simulink model "Crane_LQR_realSetup2016_obnoxious"  (R2016b)
settings: Solver=VariableStepAuto  StartTime=0.0  StopTime=30  RelTol=1e-3
undefined symbols (not defined in the file): adinchannels, adinchannelsencoders, adingain, adingainencoders, adinoffs, adinoffsencoders, Ao, Bo, Co, daoutchannels, daoutgain, daoutoffs, Discrete, Do, F, h, Humusoft, MF634, RefFWD, sigbuilder_block, Time, Ts
libraries: sldrtlib x3, dspfdesign x2, ctrlSharedLib x1
settings Model: Creator=tcbooij  LastModifiedBy=tcbooij

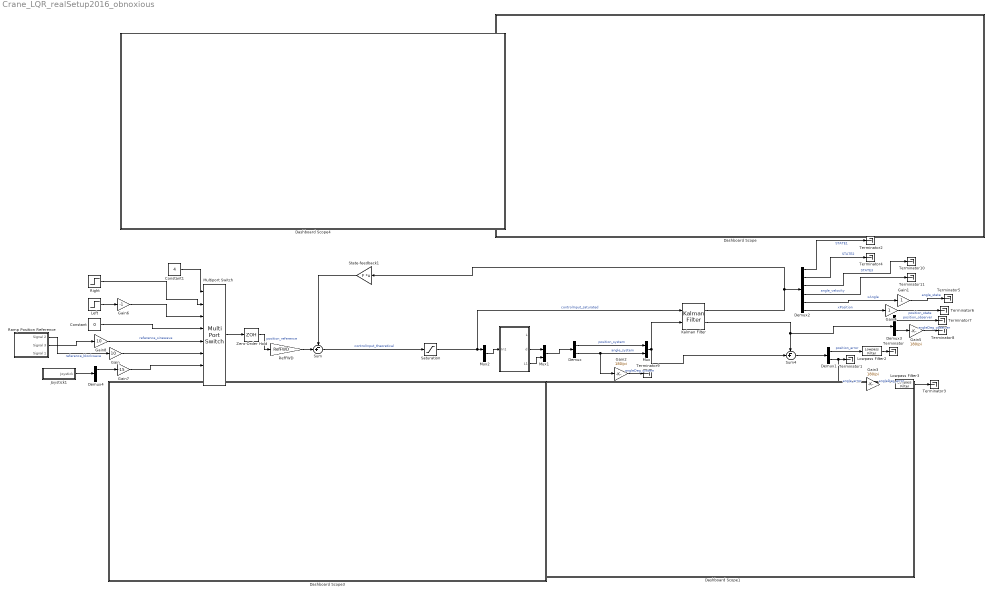
== system Crane_LQR_realSetup2016_obnoxious ==
  " " : Subsystem  LoadFcn=hwinit  InitFcn=hwinit  mask{h=h}
      mask prompts: h "Sampling period [s]"
      mask Display: disp('Crane')
  Constant : Constant  Value=0
  Constant1 : Constant  Value=4
  Dashboard Scope : Subsystem  DialogController=hmiCreateDDGDialog  IsWebBlock=on  mask(MWDashboardBlock){webBlockId=9ceaf0bf-3731-4580-b602-55a798613066, webBlockType=sdiscope, ShowInitialText=on, HMISrcModelName=Crane_LQR_realSetup2016_obnoxious}
      mask prompts: webBlockId "WebBlock Id"; webBlockType "WebBlock Type"; HMISrcModelName "Source Model"
      mask help: SimulinkHMI:dialogs:HMIScopeDialogDesc
      mask Help: helpview([docroot '/mapfiles/simulink.map'], 'hmi_scope')
      mask Display:
      | if strcmp(get_param(bdroot(gcb),'BlockDiagramType'), 'library')
      |     image([(matlabroot) '/toolbox/simulink/hmi/icons/DashboardScope.png']);
      | end
  Dashboard Scope1 : Subsystem  DialogController=hmiCreateDDGDialog  IsWebBlock=on  mask(MWDashboardBlock){webBlockId=94ce42f8-c4e1-41da-82c1-a31c02963333, webBlockType=sdiscope, ShowInitialText=on, HMISrcModelName=Crane_LQR_realSetup2016_obnoxious}
      mask prompts: webBlockId "WebBlock Id"; webBlockType "WebBlock Type"; HMISrcModelName "Source Model"
      mask help: SimulinkHMI:dialogs:HMIScopeDialogDesc
      mask Help: helpview([docroot '/mapfiles/simulink.map'], 'hmi_scope')
      mask Display:
      | if strcmp(get_param(bdroot(gcb),'BlockDiagramType'), 'library')
      |     image([(matlabroot) '/toolbox/simulink/hmi/icons/DashboardScope.png']);
      | end
  Dashboard Scope3 : Subsystem  DialogController=hmiCreateDDGDialog  IsWebBlock=on  mask(MWDashboardBlock){webBlockId=8652e169-738a-43eb-99bc-869d98056901, webBlockType=sdiscope, ShowInitialText=on, HMISrcModelName=Crane_LQR_realSetup2016_obnoxious}
      mask prompts: webBlockId "WebBlock Id"; webBlockType "WebBlock Type"; HMISrcModelName "Source Model"
      mask help: SimulinkHMI:dialogs:HMIScopeDialogDesc
      mask Help: helpview([docroot '/mapfiles/simulink.map'], 'hmi_scope')
      mask Display:
      | if strcmp(get_param(bdroot(gcb),'BlockDiagramType'), 'library')
      |     image([(matlabroot) '/toolbox/simulink/hmi/icons/DashboardScope.png']);
      | end
  Dashboard Scope4 : Subsystem  DialogController=hmiCreateDDGDialog  IsWebBlock=on  mask(MWDashboardBlock){webBlockId=041abe84-c255-4045-9a48-2957c8828250, webBlockType=sdiscope, ShowInitialText=on, HMISrcModelName=Crane_LQR_realSetup2016_obnoxious}
      mask prompts: webBlockId "WebBlock Id"; webBlockType "WebBlock Type"; HMISrcModelName "Source Model"
      mask help: SimulinkHMI:dialogs:HMIScopeDialogDesc
      mask Help: helpview([docroot '/mapfiles/simulink.map'], 'hmi_scope')
      mask Display:
      | if strcmp(get_param(bdroot(gcb),'BlockDiagramType'), 'library')
      |     image([(matlabroot) '/toolbox/simulink/hmi/icons/DashboardScope.png']);
      | end
  Demux{,1,3..4} (4 alike) : Demux  Outputs=2
  Demux2 : Demux  Outputs=6
  Gain : Gain  Gain=10
  Gain1 : Gain
  Gain2 : Gain  Gain=180/pi
  Gain3 : Gain  Gain=180/pi
  Gain4 : Gain
  Gain5 : Gain  Gain=180/pi
  Gain6 : Gain  Gain=-1
  Gain7 : Gain  Gain=-15
  Gain8 : Gain  Gain=10
  Joystick1 : Subsystem
      mask Display: disp('Joystick')
  Kalman Filter : ctrlSharedLib/Kalman Filter  TimeDomain=Discrete-Time  UseCurrentEstimator=on  ModelSource=Individual A, B, C, D matrices  ModelSourceVariable=ss(0.95,1,1,0,1)  A=Ao  B=Bo  C=Co  D=Do  NumberOfStates=1  NumberOfInputs=1  NumberOfOutputs=1  InitialEstimateSource=Dialog  X0=0  P0=10  UseK=off  UseGH=off  NumberOfProcessNoiseInputs=1  G=1  TimeInvariantG=on  H=0  TimeInvariantH=on  Q=0.1  TimeInvariantQ=on  R=[1,0;0,5]  TimeInvariantR=on  N=0  TimeInvariantN=on  AddInputPort=on  AddEnablePort=off  OutputEstimatedY=on  OutputP=off  Ts=-1
  Left : Step  Time=3  After=4  SampleTime=Ts
  Lowpass Filter2 : dspfdesign/Lowpass Filter  FilterType=IIR  DesignForMinimumOrder=on  FilterOrder=50  PassbandFrequency=5e2  StopbandFrequency=3e3  PassbandRipple=0.1  StopbandAttenuation=80  InheritSampleRate=off  SampleRate=44100  SimulateUsing=Interpreted execution  roundingMode=Floor  coeffsDataTypeStr=fixdt(1,16)
  Lowpass Filter3 : dspfdesign/Lowpass Filter  FilterType=IIR  DesignForMinimumOrder=on  FilterOrder=50  PassbandFrequency=5e2  StopbandFrequency=3e3  PassbandRipple=0.1  StopbandAttenuation=80  InheritSampleRate=off  SampleRate=44100  SimulateUsing=Interpreted execution  roundingMode=Floor  coeffsDataTypeStr=fixdt(1,16)
  Multiport Switch : MultiPortSwitch  Inputs=6  DataPortForDefault=Additional data port
  Mux : Mux  Inputs=2
  Mux1 : Mux  Inputs=2
  Mux2 : Mux  Inputs=2
  Ramp Position Reference : Subsystem  Tag=STV Subsys  LoadFcn=sigbuilder_block('load');  StartFcn=sigbuilder_block('start');  StopFcn=sigbuilder_block('stop');  ClipboardFcn=sigbuilder_block('clipboard');  mask(Sigbuilder block){tuvar=[0:10]}
      mask help: Simulink:masks:SigbuilderBlock_MD
      mask init:
      | if ~strcmp(get_param(bdroot(gcbh),'SimulationStatus'),'stopped') tuvar = sigbuilder_block('maskInit'); end
      settings: CopyFcn=sigbuilder_block('copy');  DeleteFcn=sigbuilder_block('delete');  ModelCloseFcn=sigbuilder_block('modelClose');  PreSaveFcn=sigbuilder_block('preSave');  PauseFcn=sigbuilder_block('pause');  ContinueFcn=sigbuilder_block('continue');  NameChangeFcn=sigbuilder_block('namechange');  OpenFcn=sigbuilder_block('open',[451.5 41.25 580.5 402.75 ]);  CloseFcn=sigbuilder_block('close');
      mask Display: plot(0, 0, 100, 100,[2, 2, 32, 32, 2], [68, 8, 8, 68, 68],[32, 2], [38, 38], [32, 19, 2],[53, 60, 44], [32, 17, 17, 2],[16, 16, 31, 31]);txt = getActiveGroup(gcbh);text(2, 100, txt,'verticalAlignment', 'top');
  RefFWD : Gain  Gain=RefFWD
  Right : Step  Time=3  After=6  SampleTime=Ts
  Saturation : Saturate  UpperLimit=10  LowerLimit=-10
  State-feedback1 : Gain  Gain=F  Multiplication=Matrix(K*u)
  Sum : Sum  Inputs=-+|
  Sum4 : Sum  Inputs=-+|
  Terminator{,1..11} (12 alike) : Terminator
  Zero-Order Hold : ZeroOrderHold  SampleTime=Ts
  wires:
  Demux1/2 -> Gain3/1, Terminator1/1  "angle_error"
  Demux1/1 -> Lowpass Filter2/1  "position_error"
  Gain2/1 -> Terminator9/1  "angleDeg_system"
  Gain3/1 -> Lowpass Filter3/1  "angleDeg_error"
  Demux/2 -> Gain2/1, Mux/2  "angle_system"
  Demux/1 -> Mux/1  "position_system"
  Sum/1 -> Saturation/1  "controlInput_theoretical"
  Sum4/1 -> Demux1/1
  Demux2/6 -> Gain4/1  "xPosition"
  Demux2/5 -> Gain1/1  "xAngle"
  Demux2/2 -> Terminator4/1  "STATE2"
  Demux2/1 -> Terminator2/1  "STATE1"
  Gain1/1 -> Terminator5/1  "angle_state"
  Gain4/1 -> Terminator6/1  "position_state"
  RefFWD/1 -> Sum/2
  State-feedback1/1 -> Sum/1
  Mux1/1 -> Demux/1
  " "/2(d) -> Mux1/1
  " "/3(L1) -> Mux1/2
  Mux2/1 -> " "/1(In1)
  Demux3/2 -> Gain5/1
  Demux3/1 -> Terminator7/1  "position_observer"
  Gain5/1 -> Terminator8/1  "angleDeg_observer"
  Right/1 -> Multiport Switch/2
  Multiport Switch/1 -> Zero-Order Hold/1
  Left/1 -> Gain6/1
  Gain6/1 -> Multiport Switch/3
  Constant/1 -> Multiport Switch/4
  Ramp Position Reference/1(Signal 2) -> Gain/1  "reference_blockwave"
  Joystick1/1(Joystick) -> Demux4/1
  Demux4/1 -> Gain7/1
  Constant1/1 -> Multiport Switch/1
  Zero-Order Hold/1 -> RefFWD/1  "position_reference"
  Gain/1 -> Multiport Switch/6
  Gain7/1 -> Multiport Switch/7
  Kalman Filter/1 -> State-feedback1/1, Demux2/1
  Kalman Filter/2 -> Sum4/1, Demux3/1
  Saturation/1 -> Mux2/1, Kalman Filter/1  "controlInput_saturated"
  Gain8/1 -> Multiport Switch/5  "reference_sinewave"
  Ramp Position Reference/2(Signal 3) -> Gain8/1
  Mux/1 -> Sum4/2, Kalman Filter/2
  Lowpass Filter2/1 -> Terminator/1
  Lowpass Filter3/1 -> Terminator3/1
  Demux2/3 -> Terminator10/1  "STATE3"
  Demux2/4 -> Terminator11/1  "angle_velocity"

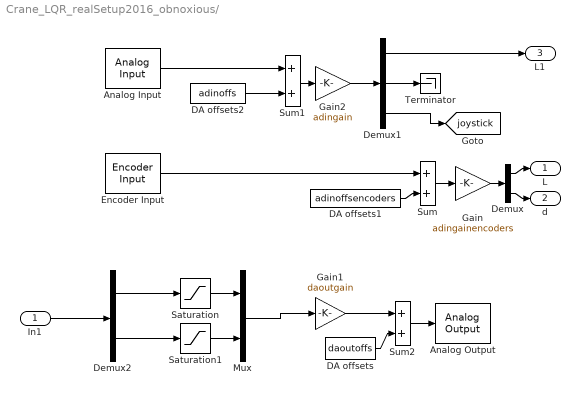
== system Crane_LQR_realSetup2016_obnoxious/  ==
  In1 : Inport
  Analog Input : sldrtlib/Analog Input  SampleTime=h  MaxMissedTicks=ticklost  ShowMissedTicks=off  YieldWhenWaiting=off  DrvName=Humusoft/MF634  DrvAddress=4294967295  DrvOptions=0  Channels=[adinchannels]  RangeMode=2  VoltRange=1  DataType=1
      settings: AttributesFormatString=Humusoft\nMF634 [auto]
  Analog Output : sldrtlib/Analog Output  SampleTime=h  MaxMissedTicks=ticklost  ShowMissedTicks=off  YieldWhenWaiting=off  DrvName=Humusoft/MF634  DrvAddress=4294967295  DrvOptions=0  Channels=[daoutchannels]  RangeMode=2  VoltRange=1  InitialValue=0  FinalValue=0
      settings: AttributesFormatString=Humusoft\nMF634 [auto]
  DA offsets : Constant  Value=daoutoffs
  DA offsets1 : Constant  Value=adinoffsencoders
  DA offsets2 : Constant  Value=adinoffs
  Demux : Demux  Outputs=2
  Demux1 : Demux  Outputs=[1 1 2]
  Demux2 : Demux  Outputs=2
  Encoder Input : sldrtlib/Encoder Input  SampleTime=h  MaxMissedTicks=ticklost  ShowMissedTicks=off  YieldWhenWaiting=off  DrvName=Humusoft/MF634  DrvAddress=4294967295  DrvOptions=0  Channels=[adinchannelsencoders]  QuadMode=3  IndexPulse=1  InputFilter=Inf  DataType=1
      settings: AttributesFormatString=Humusoft\nMF634 [auto]
  Gain : Gain  Gain=adingainencoders  SaturateOnIntegerOverflow=on  OutDataTypeStr=Inherit: Same as input  ParamDataTypeStr=Inherit: Same as input
  Gain1 : Gain  Gain=daoutgain  SaturateOnIntegerOverflow=on  OutDataTypeStr=Inherit: Same as input  ParamDataTypeStr=Inherit: Same as input
  Gain2 : Gain  Gain=adingain  SaturateOnIntegerOverflow=on  OutDataTypeStr=Inherit: Same as input  ParamDataTypeStr=Inherit: Same as input
  Mux : Mux  Inputs=2
  Saturation : Saturate  UpperLimit=10  LowerLimit=-10
  Saturation1 : Saturate  UpperLimit=10  LowerLimit=-10
  Sum : Sum  SaturateOnIntegerOverflow=on  InputSameDT=on  OutDataTypeStr=Inherit: Same as first input
  Sum1 : Sum  SaturateOnIntegerOverflow=on  InputSameDT=on  OutDataTypeStr=Inherit: Same as first input
  Sum2 : Sum  SaturateOnIntegerOverflow=on  InputSameDT=on  OutDataTypeStr=Inherit: Same as first input
  Terminator : Terminator
  L : Outport  Tag=Position
  d : Outport  Tag=Cable length  Port=2
  L1 : Outport  Tag=Position  Port=3
  tag scope: joystick=global
  wires:
  Gain/1 -> Demux/1
  Sum/1 -> Gain/1
  DA offsets1/1 -> Sum/2
  Sum1/1 -> Gain2/1
  Analog Input/1 -> Sum1/1
  DA offsets2/1 -> Sum1/2
  Demux/1 -> L/1
  Demux/2 -> d/1
  Gain2/1 -> Demux1/1
  Demux1/3 -> [joystick]
  Demux1/1 -> L1/1
  Gain1/1 -> Sum2/1
  Sum2/1 -> Analog Output/1
  DA offsets/1 -> Sum2/2
  Encoder Input/1 -> Sum/1
  In1/1 -> Demux2/1
  Demux2/1 -> Saturation/1
  Demux2/2 -> Saturation1/1
  Saturation/1 -> Mux/1
  Mux/1 -> Gain1/1
  Saturation1/1 -> Mux/2
  Demux1/2 -> Terminator/1

== system Crane_LQR_realSetup2016_obnoxious/Dashboard Scope ==

== system Crane_LQR_realSetup2016_obnoxious/Dashboard Scope1 ==

== system Crane_LQR_realSetup2016_obnoxious/Dashboard Scope3 ==

== system Crane_LQR_realSetup2016_obnoxious/Dashboard Scope4 ==

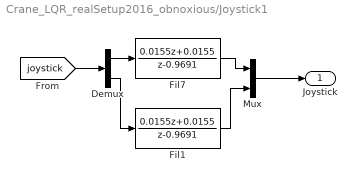
== system Crane_LQR_realSetup2016_obnoxious/Joystick1 ==
  Demux : Demux  Outputs=2
  Fil1 : DiscreteTransferFcn  Numerator=[0.0155 0.0155]  Denominator=[1 -0.9691]  SampleTime=h
  Fil7 : DiscreteTransferFcn  Numerator=[0.0155 0.0155]  Denominator=[1 -0.9691]  SampleTime=h
  Mux : Mux  Inputs=2
  Joystick : Outport
  wires:
  Mux/1 -> Joystick/1
  Fil1/1 -> Mux/2
  Demux/2 -> Fil1/1
  Demux/1 -> Fil7/1
  [joystick] -> Demux/1
  Fil7/1 -> Mux/1

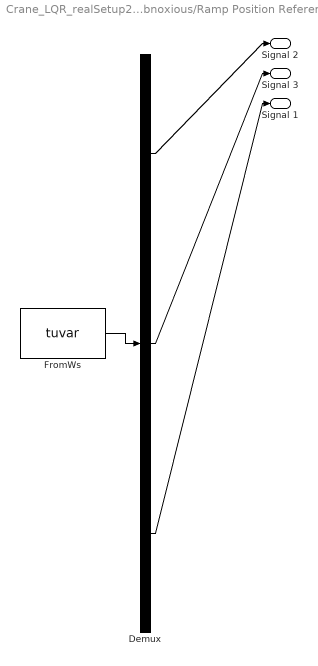
== system Crane_LQR_realSetup2016_obnoxious/Ramp Position Reference ==
  Demux : Demux  Tag=STV Demux  Outputs=3
  FromWs : FromWorkspace  Tag=STV FromWs  VariableName=tuvar  SampleTime=0
      SigBuilderData=|
      | common.afterFinalStr = 'Extrapolate'
      | common.sampleTime = 0
      | dataSet.timeRange = [0 30]
      | dataSet.name = 'Group 1'
      | sbobj.Groups.Name = 'Group 1'
      | sbobj.Groups.Signals(1).Name = 'Signal 2'
      | sbobj.Groups.Signals(1).XData = [0 2.5 5 7.5 10 12.5 15 17.5 20 22.5 25 27.5 30]
      | sbobj.Groups.Signals(1).YData = [0 0 1 1 0 0 -1 -1 0 0 1 1 0]
      | sbobj.Groups.Signals(2).Name = 'Signal 3'
      | sbobj.Groups.Signals(2).XData = [0 0.10101010101 0.20202020202 0.30303030303 0.40404040404 0.505050505051 0.606060606061 0.707070707071 0.808080808081 0.909090909091 1.0101010101 1.11111111111 ... (298 elements, 1x298)]
      | sbobj.Groups.Signals(2).YData = [0 0.0634239196566 0.126592453574 0.18925124436 0.251147987181 0.312033445698 0.37166245566 0.429794912089 0.4861967361 0.540640817456 0.592907929055 0.642787609687 ... (298 elements, 1x298)]
      | sbobj.Groups.Signals(3).Name = 'Signal 1'
      | sbobj.Groups.Signals(3).XData = [0 0.020202020202 0.040404040404 0.0606060606061 0.0808080808081 0.10101010101 0.121212121212 0.141414141414 0.161616161616 0.181818181818 0.20202020202 0.222222222222 ... (1486 elements, 1x1486)]
      | sbobj.Groups.Signals(3).YData = [0 0.0634239196566 0.126592453574 0.18925124436 0.251147987181 0.312033445698 0.37166245566 0.429794912089 0.4861967361 0.540640817456 0.592907929055 0.642787609687 ... (1486 elements, 1x1486)]
      | sbobj.Groups.TimeRange = [0 30]
  Signal 2 : Outport  Tag=STV Outport
  Signal 3 : Outport  Tag=STV Outport  Port=2
  Signal 1 : Outport  Tag=STV Outport  Port=3
  wires:
  FromWs/1 -> Demux/1
  Demux/1 -> Signal 2/1
  Demux/2 -> Signal 3/1
  Demux/3 -> Signal 1/1
